simulink subsystem "D1Szakaszteljes"  (R2024b)
settings: Solver=VariableStepAuto  StartTime=0.0  StopTime=10.0  RelTol=1e-3
settings Model: Creator=Asus  LastModifiedBy=Asus

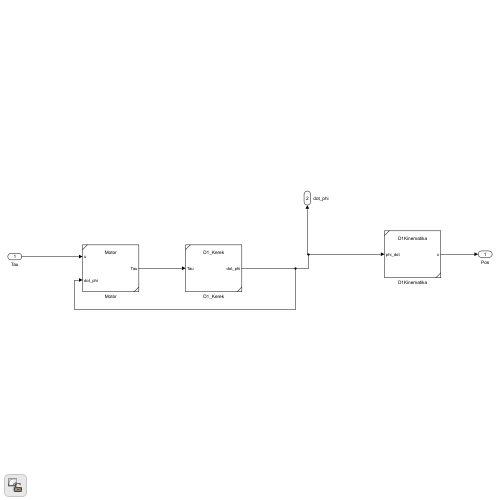
[thumbnail: Simulink's stored preview of the top-level diagram]
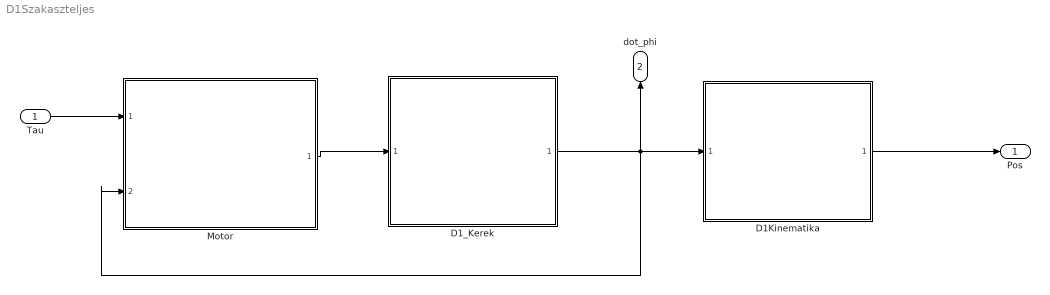
== system D1Szakaszteljes ==
  Tau : Inport
  D1Kinematika : Subsystem  ReferencedSubsystem=D1Kinematika
  D1_Kerek : Subsystem  ReferencedSubsystem=D1_Kerek
  Motor : Subsystem  ReferencedSubsystem=Motor
  Pos : Outport
  dot_phi : Outport  Port=2
  wires:
  Tau/1 -> Motor/1
  D1Kinematika/1 -> Pos/1
  Motor/1 -> D1_Kerek/1
  D1_Kerek/1 -> dot_phi/1, D1Kinematika/1, Motor/2
